simulink model "s_hover_lqr"  (Simulink 8.0)
settings: Solver=ode4  StartTime=0.0  StopTime=20  FixedStep=0.001  RelTol=1e-3
values from neighbouring files (symbols this model uses):
  CMD_RATE_LIMIT = 1    [setup_lab_hover.m]
  K = zeros(4,6)    [setup_lab_hover.m]
  K_AMP = 3    [setup_lab_hover.m]
  V_bias = 5.0    (= 5)    [setup_lab_hover.m]
  VMAX_AMP = 12    [setup_lab_hover.m]
  VMAX_DAC = 10    [setup_lab_hover.m]
  wcf = 2 * pi * 20    (= 125.663706144)    [setup_lab_hover.m]
  zetaf = 0.6    [setup_lab_hover.m]
undefined symbols (not defined in the file or in its folder): A, AMIO, B, BMIO, C, CMIO, D, DMIO, KMIO
libraries: simulink_extras x7
settings Model: Creator=hpineros  LastModifiedBy=David  ExtModeTrigDuration=10000  TunableVars=A,B,C,CMD_RATE_LIMIT,D,INT_JOYSTICK_SAT_LOWER,INT_JOYSTICK_SAT_UPPER,JOYSTICK_X_DZ,JOYSTICK_Y_DZ,Jp,Jr,Jy,K,K_AMP,K_EC_P,K_EC_R,K_EC_Y,K_JOYSTICK_X,K_JOYSTICK_Y,Kf,Ktc,Ktn,Q,R,VMAX_AMP,VMAX_DAC,V_bias,g,l,wcf,zetaf  TunableVarsStorageClass=Auto,Auto,Auto,Auto,Auto,Auto,Auto,Auto,Auto,Auto,Auto,Auto,Auto,Auto,Auto,Auto,Auto,Auto,Auto,Auto,Auto,Auto,Auto,Auto,Auto,Auto,Auto,Auto,Auto,Auto,Auto  TunableVarsTypeQualifier=,,,,,,,,,,,,,,,,,,,,,,,,,,,,,,
settings SolverCC: PositivePriorityOrder=on
settings DataIOCC: SignalLoggingSaveFormat=ModelDataLogs
settings OptimizationCC: InlineParams=on  InitFltsAndDblsToZero=on
settings DebuggingCC: SaveWithParameterizedLinksMsg=none  FcnCallInpInsideContextMsg=UseLocalSettings  StrictBusMsg=Warning
settings RTWCC: SystemTargetFile=quarc_windows.tlc  TemplateMakefile=quarc_default_tmf  Description=QuaRC Win32 Target  ProcessScript=quarc_windows_make_rtw_hook
settings STFCustomTargetCC: TargetFcnLib=ansi_tfl_tmw.mat  TargetPreCompLibLocation=C:\PROGRA~2\QUARC\lib\2011a\windows\release  CodeReplacementLibrary=ANSI_C  GeneratePreprocessorConditionals=Disable all  SystemTargetFile=quarc_windows.tlc
settings GRTTargetCC: TargetFcnLib=ansi_tfl_tmw.mat  TargetPreCompLibLocation=C:\PROGRA~2\QUARC\lib\2011a\windows\release  ParMdlRefBuildCompliant=off  CompOptLevelCompliant=off  ConcurrentExecutionCompliant=off  CombineOutputUpdateFcns=off  MatFileLogging=off  GRTInterface=on  ExtMode=on  ExtModeMexFile=quarc_comm

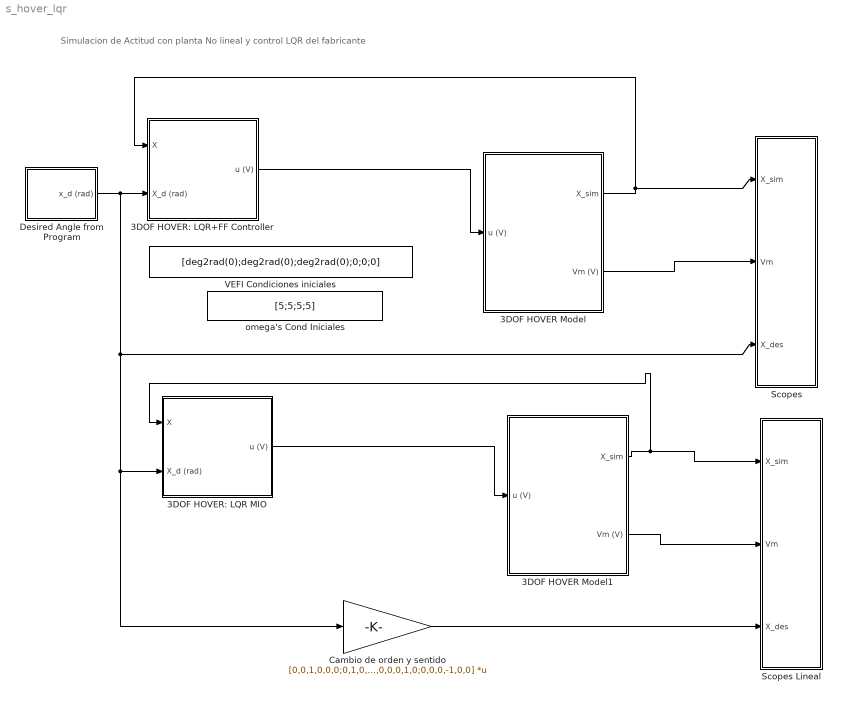
== system s_hover_lqr ==
  note: Simulacion de Actitud con planta No lineal y control LQR del fabricante
  3DOF HOVER Model : Subsystem
  3DOF HOVER Model1 : Subsystem
  3DOF HOVER: LQR MIO : Subsystem
  3DOF HOVER: LQR+FF Controller : Subsystem
  Cambio de orden y sentido : Gain  Gain=[0,0,1,0,0,0;0,1,0,0,0,0;-1,0,0,0,0,0;0,0,0,0,0,1;0,0,0,0,1,0;0,0,0,-1,0,0]  Multiplication=Matrix(K*u)
  Desired Angle from Program : Subsystem
  Scopes : Subsystem
  Scopes Lineal : Subsystem
  VEFI Condiciones iniciales : Constant  Value=[deg2rad(0);deg2rad(0);deg2rad(0);0;0;0]
  omega's Cond Iniciales : Constant  Value=[5;5;5;5]
  wires:
  Desired Angle from Program/1(x_d (rad)) -> 3DOF HOVER: LQR+FF Controller/2(X_d (rad)), Scopes/3(X_des), 3DOF HOVER: LQR MIO/2(X_d (rad)), Cambio de orden y sentido/1
  3DOF HOVER: LQR+FF Controller/1(u (V)) -> 3DOF HOVER Model/1(u (V))
  3DOF HOVER Model/1(X_sim) -> Scopes/1(X_sim), 3DOF HOVER: LQR+FF Controller/1(X)
  3DOF HOVER Model1/1(X_sim) -> Scopes Lineal/1(X_sim), 3DOF HOVER: LQR MIO/1(X)
  3DOF HOVER Model1/2(Vm (V)) -> Scopes Lineal/2(Vm)
  3DOF HOVER: LQR MIO/1(u (V)) -> 3DOF HOVER Model1/1(u (V))
  3DOF HOVER Model/2(Vm (V)) -> Scopes/2(Vm)
  Cambio de orden y sentido/1 -> Scopes Lineal/3(X_des)

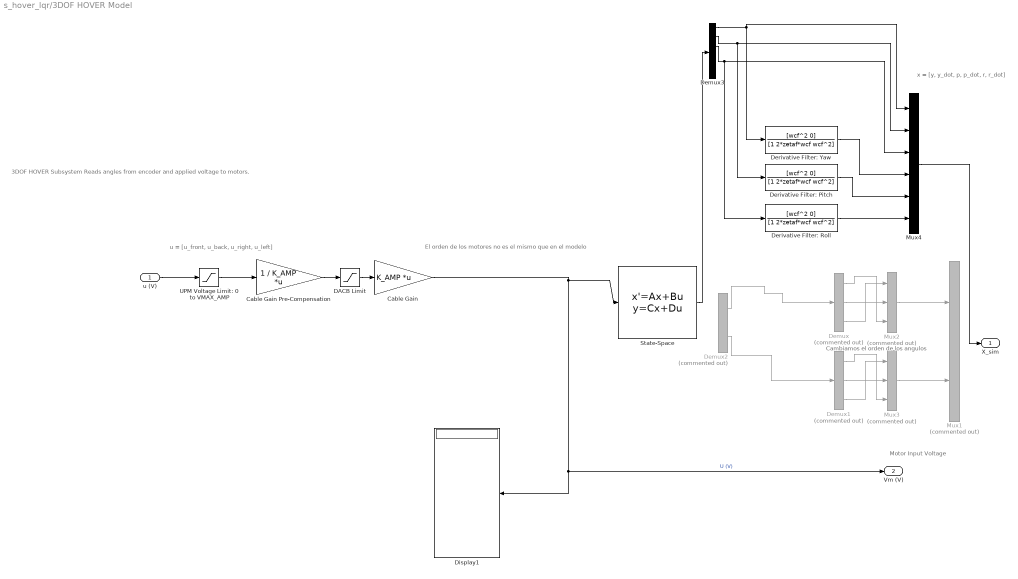
== system s_hover_lqr/3DOF HOVER Model ==
  note: Cambiamos el orden de los angulos
  note: 3DOF HOVER Subsystem
      | Reads angles from encoder and applied voltage to motors.
  note: Motor Input Voltage
  note: u = [u_front, u_back, u_right, u_left]
  note: El orden de los motores no es el mismo que en el modelo
  note: x = [y, y_dot, p, p_dot, r, r_dot]
  u (V) : Inport
  Cable Gain : Gain  Gain=K_AMP  Multiplication=Matrix(K*u)  SaturateOnIntegerOverflow=on  OutDataTypeStr=Inherit: Same as input  ParamDataTypeStr=Inherit: Same as input
  Cable Gain Pre-Compensation : Gain  Gain=1 / K_AMP  Multiplication=Matrix(K*u)  SaturateOnIntegerOverflow=on  OutDataTypeStr=Inherit: Same as input  ParamDataTypeStr=Inherit: Same as input
  DACB Limit : Saturate  UpperLimit=VMAX_DAC  LowerLimit=-VMAX_DAC
  Demux : Demux  Commented=on  Outputs=3
  Demux1 : Demux  Commented=on  Outputs=3
  Demux2 : Demux  Commented=on  Outputs=2
  Demux3 : Demux  Outputs=[1 1 1 1 1 1]
  Derivative Filter: Pitch : TransferFcn  Numerator=[wcf^2 0]  Denominator=[1 2*zetaf*wcf wcf^2]
  Derivative Filter: Roll : TransferFcn  Numerator=[wcf^2 0]  Denominator=[1 2*zetaf*wcf wcf^2]
  Derivative Filter: Yaw : TransferFcn  Numerator=[wcf^2 0]  Denominator=[1 2*zetaf*wcf wcf^2]
  Display1 : Display
  Mux1 : Mux  Commented=on  Inputs=2
  Mux2 : Mux  Commented=on  Inputs=3
  Mux3 : Mux  Commented=on  Inputs=3
  Mux4 : Mux  Inputs=6
  State-Space : StateSpace  A=A  B=B  C=C  D=D  X0=[deg2rad(0);deg2rad(0);deg2rad(0);0;0;0]
  UPM Voltage Limit: 0 to VMAX_AMP : Saturate  UpperLimit=VMAX_AMP  LowerLimit=0
  X_sim : Outport
  Vm (V) : Outport  Port=2
  wires:
  Cable Gain/1 -> Vm (V)/1, Display1/1, State-Space/1  "U (V)"
  DACB Limit/1 -> Cable Gain/1
  u (V)/1 -> UPM Voltage Limit: 0 to VMAX_AMP/1
  UPM Voltage Limit: 0 to VMAX_AMP/1 -> Cable Gain Pre-Compensation/1
  Cable Gain Pre-Compensation/1 -> DACB Limit/1
  Demux2/1 -> Demux/1
  Demux2/2 -> Demux1/1
  Demux/2 -> Mux2/2
  Demux/3 -> Mux2/1
  Demux/1 -> Mux2/3
  Demux1/2 -> Mux3/2
  Demux1/3 -> Mux3/1
  Demux1/1 -> Mux3/3
  Mux3/1 -> Mux1/2
  Mux2/1 -> Mux1/1
  Demux3/3 -> Derivative Filter: Roll/1, Mux4/3
  Demux3/2 -> Derivative Filter: Pitch/1, Mux4/2
  Derivative Filter: Roll/1 -> Mux4/6
  Derivative Filter: Pitch/1 -> Mux4/5
  Derivative Filter: Yaw/1 -> Mux4/4
  Demux3/1 -> Mux4/1, Derivative Filter: Yaw/1
  State-Space/1 -> Demux3/1
  Mux4/1 -> X_sim/1

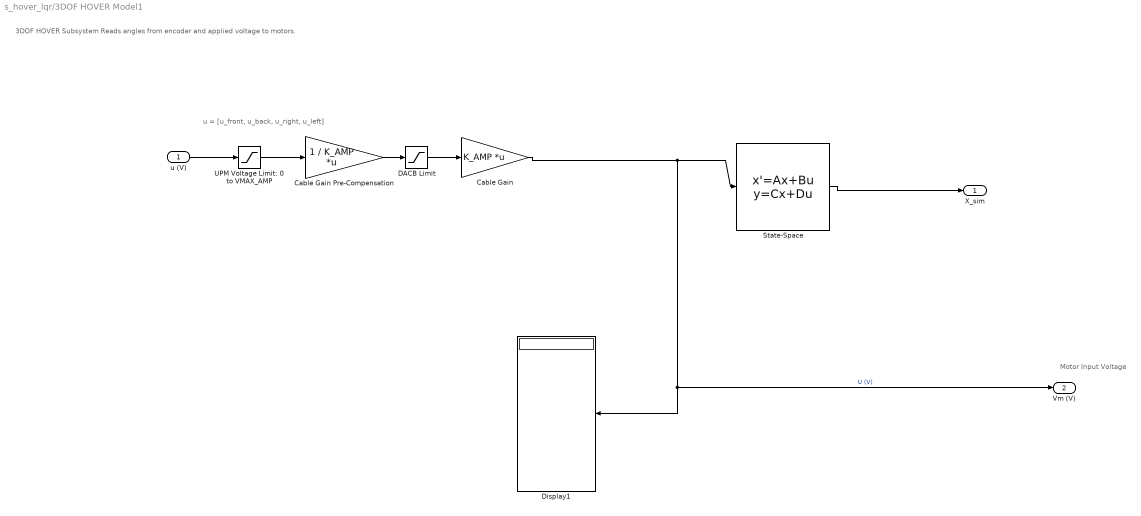
== system s_hover_lqr/3DOF HOVER Model1 ==
  note: 3DOF HOVER Subsystem
      | Reads angles from encoder and applied voltage to motors.
  note: Motor Input Voltage
  note: u = [u_front, u_back, u_right, u_left]
  u (V) : Inport
  Cable Gain : Gain  Gain=K_AMP  Multiplication=Matrix(K*u)  SaturateOnIntegerOverflow=on  OutDataTypeStr=Inherit: Same as input  ParamDataTypeStr=Inherit: Same as input
  Cable Gain Pre-Compensation : Gain  Gain=1 / K_AMP  Multiplication=Matrix(K*u)  SaturateOnIntegerOverflow=on  OutDataTypeStr=Inherit: Same as input  ParamDataTypeStr=Inherit: Same as input
  DACB Limit : Saturate  UpperLimit=VMAX_DAC  LowerLimit=-VMAX_DAC
  Display1 : Display
  State-Space : StateSpace  A=AMIO  B=BMIO  C=CMIO  D=DMIO  X0=[deg2rad(0);deg2rad(0);deg2rad(0);0;0;0]
  UPM Voltage Limit: 0 to VMAX_AMP : Saturate  UpperLimit=VMAX_AMP  LowerLimit=0
  X_sim : Outport
  Vm (V) : Outport  Port=2
  wires:
  Cable Gain/1 -> Vm (V)/1, Display1/1, State-Space/1  "U (V)"
  DACB Limit/1 -> Cable Gain/1
  u (V)/1 -> UPM Voltage Limit: 0 to VMAX_AMP/1
  UPM Voltage Limit: 0 to VMAX_AMP/1 -> Cable Gain Pre-Compensation/1
  Cable Gain Pre-Compensation/1 -> DACB Limit/1
  State-Space/1 -> X_sim/1

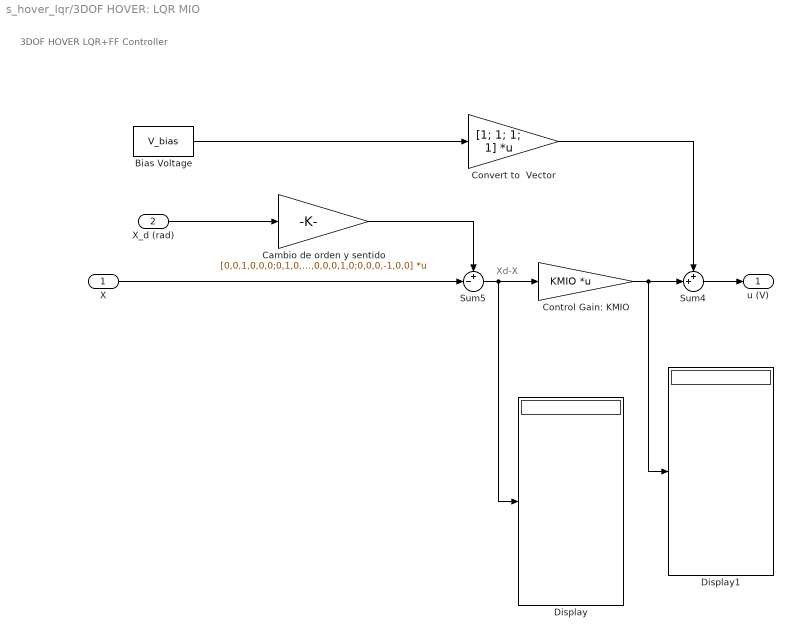
== system s_hover_lqr/3DOF HOVER: LQR MIO ==
  note: Xd-X
  note: 3DOF HOVER LQR+FF Controller
  X : Inport
  X_d (rad) : Inport  Port=2
  Bias Voltage : Constant  Value=V_bias
  Cambio de orden y sentido : Gain  Gain=[0,0,1,0,0,0;0,1,0,0,0,0;-1,0,0,0,0,0;0,0,0,0,0,1;0,0,0,0,1,0;0,0,0,-1,0,0]  Multiplication=Matrix(K*u)
  Control Gain: KMIO : Gain  Gain=KMIO  Multiplication=Matrix(K*u) (u vector)
  Convert to  Vector : Gain  Gain=[1; 1; 1; 1]  Multiplication=Matrix(K*u)
  Display : Display
  Display1 : Display
  Sum4 : Sum  Inputs=++|
  Sum5 : Sum  Inputs=+-|
  u (V) : Outport
  wires:
  Sum5/1 -> Control Gain: KMIO/1, Display/1
  X_d (rad)/1 -> Cambio de orden y sentido/1
  Convert to  Vector/1 -> Sum4/1
  Control Gain: KMIO/1 -> Sum4/2, Display1/1
  Bias Voltage/1 -> Convert to  Vector/1
  Sum4/1 -> u (V)/1
  X/1 -> Sum5/2
  Cambio de orden y sentido/1 -> Sum5/1

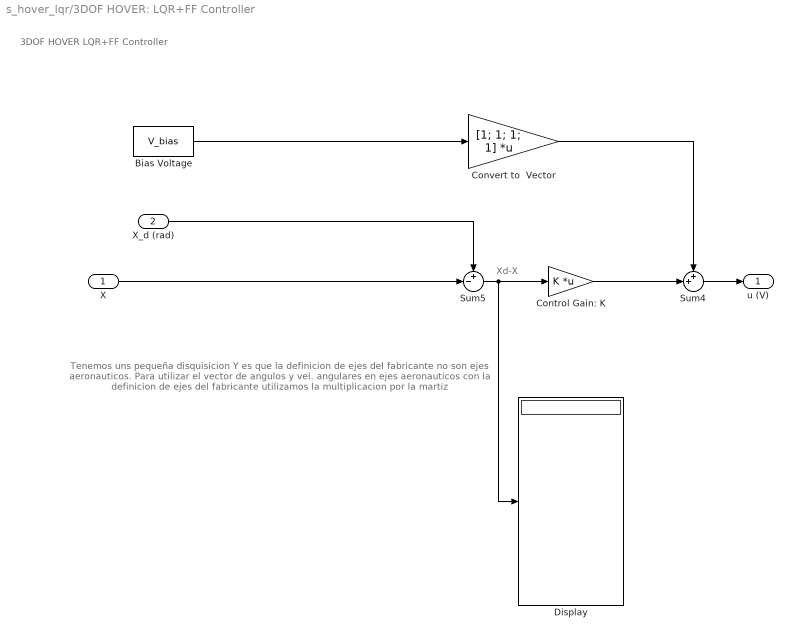
== system s_hover_lqr/3DOF HOVER: LQR+FF Controller ==
  note: Xd-X
  note: 3DOF HOVER LQR+FF Controller
  note: Tenemos uns pequeña disquisicion
      | Y es que la definicion de ejes del fabricante no son ejes aeronauticos.
      | Para utilizar el vector de angulos y vel. angulares en ejes aeronauticos
      | con la definicion de ejes del fabricante utilizamos la multiplicacion por la martiz
  X : Inport
  X_d (rad) : Inport  Port=2
  Bias Voltage : Constant  Value=V_bias
  Control Gain: K : Gain  Gain=K  Multiplication=Matrix(K*u)
  Convert to  Vector : Gain  Gain=[1; 1; 1; 1]  Multiplication=Matrix(K*u)
  Display : Display
  Sum4 : Sum  Inputs=++|
  Sum5 : Sum  Inputs=+-|
  u (V) : Outport
  wires:
  Sum5/1 -> Control Gain: K/1, Display/1
  X_d (rad)/1 -> Sum5/1
  Convert to  Vector/1 -> Sum4/1
  Control Gain: K/1 -> Sum4/2
  Bias Voltage/1 -> Convert to  Vector/1
  Sum4/1 -> u (V)/1
  X/1 -> Sum5/2

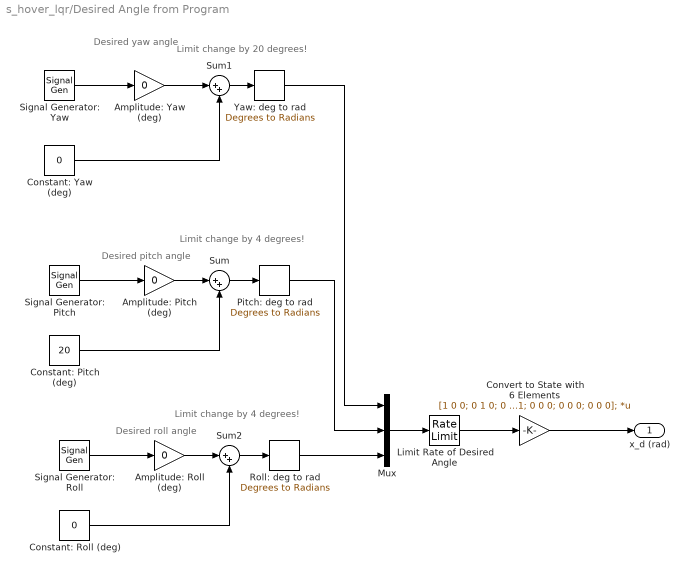
== system s_hover_lqr/Desired Angle from Program ==
  note: Limit change by
      | 4 degrees!
  note: Limit change by
      | 20 degrees!
  note: Limit change by
      | 4 degrees!
  note: Desired roll angle
  note: Desired pitch angle
  note: Desired yaw angle
  Amplitude: Pitch (deg) : Gain  Gain=0
  Amplitude: Roll (deg) : Gain  Gain=0
  Amplitude: Yaw (deg) : Gain  Gain=0
  Constant: Pitch (deg) : Constant  Value=20
  Constant: Roll (deg) : Constant  Value=0
  Constant: Yaw (deg) : Constant  Value=0
  Convert to State with 6 Elements : Gain  Gain=[1 0 0; 0 1 0; 0 0 1; 0 0 0; 0 0 0; 0 0 0];  Multiplication=Matrix(K*u)
  Limit Rate of Desired Angle : RateLimiter  RisingSlewLimit=CMD_RATE_LIMIT  FallingSlewLimit=-CMD_RATE_LIMIT
  Mux : Mux  Inputs=3
  Pitch: deg to rad : simulink_extras/Transformations/Degrees to Radians
  Roll: deg to rad : simulink_extras/Transformations/Degrees to Radians
  Signal Generator: Pitch : SignalGenerator  WaveForm=square  Frequency=0.0000001
  Signal Generator: Roll : SignalGenerator  WaveForm=square  Frequency=0.08
  Signal Generator: Yaw : SignalGenerator  WaveForm=square  Frequency=0.04
  Sum : Sum  Inputs=|++
  Sum1 : Sum  Inputs=|++
  Sum2 : Sum  Inputs=|++
  Yaw: deg to rad : simulink_extras/Transformations/Degrees to Radians
  x_d (rad) : Outport
  wires:
  Convert to State with 6 Elements/1 -> x_d (rad)/1
  Limit Rate of Desired Angle/1 -> Convert to State with 6 Elements/1
  Roll: deg to rad/1 -> Mux/3
  Pitch: deg to rad/1 -> Mux/2
  Yaw: deg to rad/1 -> Mux/1
  Sum2/1 -> Roll: deg to rad/1
  Signal Generator: Roll/1 -> Amplitude: Roll (deg)/1
  Amplitude: Roll (deg)/1 -> Sum2/1
  Constant: Roll (deg)/1 -> Sum2/2
  Sum/1 -> Pitch: deg to rad/1
  Signal Generator: Pitch/1 -> Amplitude: Pitch (deg)/1
  Amplitude: Pitch (deg)/1 -> Sum/1
  Constant: Pitch (deg)/1 -> Sum/2
  Sum1/1 -> Yaw: deg to rad/1
  Signal Generator: Yaw/1 -> Amplitude: Yaw (deg)/1
  Amplitude: Yaw (deg)/1 -> Sum1/1
  Constant: Yaw (deg)/1 -> Sum1/2
  Mux/1 -> Limit Rate of Desired Angle/1

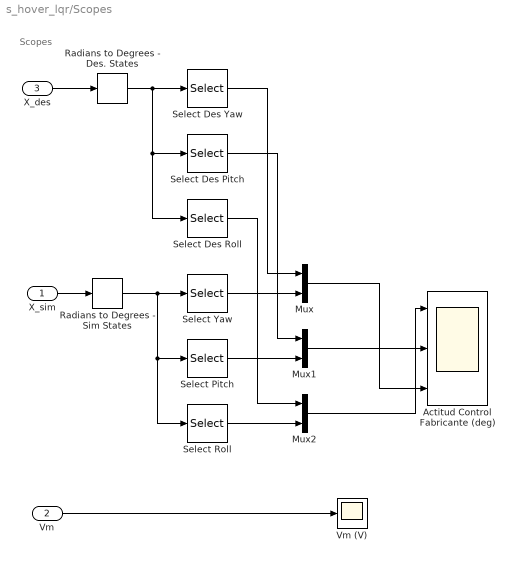
== system s_hover_lqr/Scopes ==
  note: Scopes
  X_sim : Inport
  Vm : Inport  Port=2
  X_des : Inport  Port=3
  Actitud Control Fabricante (deg) : Scope  NumInputPorts=3
      settings: TickLabels=on  TimeRange=20  YMin=0~0~0  YMax=1.4e-008~20~0.0008  SaveName=Ensayo1
  Mux : Mux  Inputs=2
  Mux1 : Mux  Inputs=2
  Mux2 : Mux  Inputs=2
  Radians to Degrees - Des. States : simulink_extras/Transformations/Radians to Degrees
  Radians to Degrees - Sim States : simulink_extras/Transformations/Radians to Degrees
  Select Des Pitch : Selector  InputPortWidth=6  IndexOptions=Index vector (dialog)  Indices=2  OutputSizes=1
  Select Des Roll : Selector  InputPortWidth=6  IndexOptions=Index vector (dialog)  Indices=3  OutputSizes=1
  Select Des Yaw : Selector  InputPortWidth=6  IndexOptions=Index vector (dialog)  Indices=1  OutputSizes=1
  Select Pitch : Selector  InputPortWidth=6  IndexOptions=Index vector (dialog)  Indices=2  OutputSizes=1
  Select Roll : Selector  InputPortWidth=6  IndexOptions=Index vector (dialog)  Indices=3  OutputSizes=1
  Select Yaw : Selector  InputPortWidth=6  IndexOptions=Index vector (dialog)  Indices=1  OutputSizes=1
  Vm (V) : Scope
      settings: TickLabels=on  TimeRange=20  YMin=0  YMax=25  SaveName=ScopeData4
  wires:
  Select Des Roll/1 -> Mux2/1
  Select Des Pitch/1 -> Mux1/1
  Select Des Yaw/1 -> Mux/1
  Radians to Degrees - Des. States/1 -> Select Des Roll/1, Select Des Pitch/1, Select Des Yaw/1
  Select Roll/1 -> Mux2/2
  Select Pitch/1 -> Mux1/2
  Select Yaw/1 -> Mux/2
  Radians to Degrees - Sim States/1 -> Select Roll/1, Select Pitch/1, Select Yaw/1
  Vm/1 -> Vm (V)/1
  X_sim/1 -> Radians to Degrees - Sim States/1
  X_des/1 -> Radians to Degrees - Des. States/1
  Mux/1 -> Actitud Control Fabricante (deg)/3
  Mux2/1 -> Actitud Control Fabricante (deg)/1
  Mux1/1 -> Actitud Control Fabricante (deg)/2

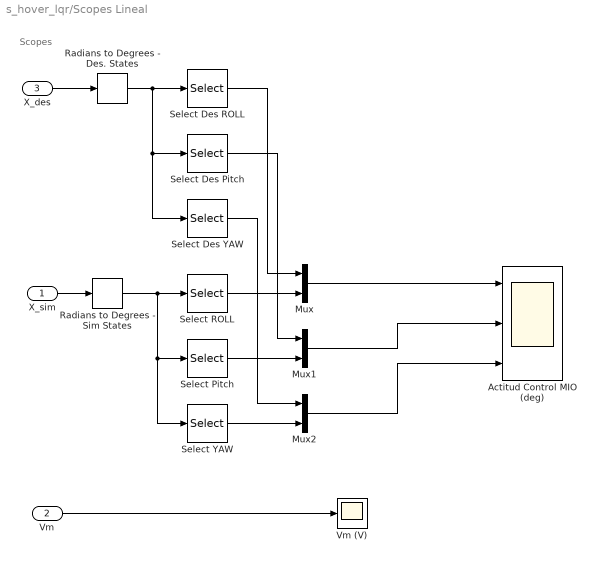
== system s_hover_lqr/Scopes Lineal ==
  note: Scopes
  X_sim : Inport
  Vm : Inport  Port=2
  X_des : Inport  Port=3
  Actitud Control MIO (deg) : Scope  NumInputPorts=3
      settings: TickLabels=on  TimeRange=20  YMin=0~-0~-0.00175  YMax=0.00055~20~0  SaveName=Ensayo1
  Mux : Mux  Inputs=2
  Mux1 : Mux  Inputs=2
  Mux2 : Mux  Inputs=2
  Radians to Degrees - Des. States : simulink_extras/Transformations/Radians to Degrees
  Radians to Degrees - Sim States : simulink_extras/Transformations/Radians to Degrees
  Select Des Pitch : Selector  InputPortWidth=6  IndexOptions=Index vector (dialog)  Indices=2  OutputSizes=1
  Select Des ROLL : Selector  InputPortWidth=6  IndexOptions=Index vector (dialog)  Indices=1  OutputSizes=1
  Select Des YAW : Selector  InputPortWidth=6  IndexOptions=Index vector (dialog)  Indices=3  OutputSizes=1
  Select Pitch : Selector  InputPortWidth=6  IndexOptions=Index vector (dialog)  Indices=2  OutputSizes=1
  Select ROLL : Selector  InputPortWidth=6  IndexOptions=Index vector (dialog)  Indices=1  OutputSizes=1
  Select YAW : Selector  InputPortWidth=6  IndexOptions=Index vector (dialog)  Indices=3  OutputSizes=1
  Vm (V) : Scope
      settings: TickLabels=on  TimeRange=20  YMin=0  YMax=25  SaveName=ScopeData4
  wires:
  Select Des YAW/1 -> Mux2/1
  Select Des Pitch/1 -> Mux1/1
  Select Des ROLL/1 -> Mux/1
  Radians to Degrees - Des. States/1 -> Select Des YAW/1, Select Des Pitch/1, Select Des ROLL/1
  Select YAW/1 -> Mux2/2
  Select Pitch/1 -> Mux1/2
  Select ROLL/1 -> Mux/2
  Radians to Degrees - Sim States/1 -> Select YAW/1, Select Pitch/1, Select ROLL/1
  Vm/1 -> Vm (V)/1
  X_sim/1 -> Radians to Degrees - Sim States/1
  X_des/1 -> Radians to Degrees - Des. States/1
  Mux/1 -> Actitud Control MIO (deg)/1
  Mux1/1 -> Actitud Control MIO (deg)/2
  Mux2/1 -> Actitud Control MIO (deg)/3
